simulink model "TxSteering_RxMVDR_4x4_HDL_IQ"  (R2023a)
settings: Solver=FixedStepDiscrete  StartTime=0.0  StopTime=stoptime  RelTol=1e-3
PreLoadFcn:
  | model_init
InitFcn:
  | model_init
model workspace (MAT data in the model file):
  socvcb : containers.Map (value not decoded)
values from neighbouring files (symbols this model uses):
  diagLoading = 5e-3    (= 0.005)    [model_init.m]
  dmaFIFOLength = 2^nextpow2(testSrc1.FrameLength*testSrc1.SamplesPerSymbol*2)    [model_init.m]
  fc = ConverterSampleRate*7/16    (= 860160000)    [model_init.m]
  FPGAClkRate = DataSampleRate/VectorSamplingFactor    (= 245760000)    [model_init.m]
  movavg_bitshift = nextpow2(windowSize)    [model_init.m]
  mvdrPipelineDelay = covMatDelay+movAvgDelay+matrixSolveDelay+normResponseDelay    [model_init.m]
  NCO_bits = 14    [model_init.m]
  numArrayElements = 4    [model_init.m]
  NumChan = 4    [model_init.m]
  reciprocalDelay = nextpow2(reciprocalin_dt.WordLength) + 1 + reciprocalin_dt.WordLength + 2      - strcmp(reciprocalin_dt.Signedness,'Signed') + 7    [model_init.m]
  rx_mag_delay = input_dt.WordLength + 2 + ceil(log2(NumChan)) + 1 + rx_mag_window_size    [model_init.m]
  rx_mag_inverse_delay = nextpow2(rx_mag_dt.WordLength) + 1 + rx_mag_dt.WordLength + 2 + 7    [model_init.m]
  rx_mag_sum_growth = nextpow2(rx_mag_window_size)    [model_init.m]
  rx_mag_window_size = 256    [model_init.m]
  s2mmFrameSize = testSrc1.FrameLength*testSrc1.SamplesPerSymbol*3    [model_init.m]
  testSrc1 = struct()    [model_init.m]
  testSrc2 = struct()    [model_init.m]
  windowSize = 4096    [model_init.m]
undefined symbols (not defined in the file or in its folder): Add, j, NumBits1, NumBits2, physconst, Shift
libraries: hdlsllib x29, simulink x15, embreciprocals x2, dspsrcs4 x2, dsphdlmathfun2 x1, embsystolicmatrixops x1, dsphdlsigops2 x1, commrfcorlib x1
(part 2 of 3)

== system TxSteering_RxMVDR_4x4_HDL_IQ/DUT/Rx Beamforming/MVDR HDL ==
  data_bus_in : Inport
  steering_vector : Inport  Port=2
  diag_loading : Inport  Port=3
  Compute Weight Vector : Subsystem
  Diagonal Loading : Subsystem
  Form Beam : Subsystem
  Form Covariance Matrix : Subsystem
  From Data Bus1 : Subsystem
  Moving Average : Subsystem
  Normalize Response : Subsystem
  data_bus_out : Outport
  computed_weights : Outport  Port=2
  wires:
  Normalize Response/2(wOut) -> Form Beam/3(weights), computed_weights/1
  Form Covariance Matrix/2(validOut) -> Moving Average/2(validIn)
  Compute Weight Vector/1(w) -> Normalize Response/1(wIn)
  steering_vector/1 -> Compute Weight Vector/3(steeringVector), Normalize Response/3(steeringVector)
  Form Covariance Matrix/1(dataOut) -> Moving Average/1(dataIn)
  Compute Weight Vector/2(validOut) -> Normalize Response/2(validIn)
  From Data Bus1/1(data) -> Form Covariance Matrix/1(dataIn)
  From Data Bus1/2(valid) -> Form Covariance Matrix/2(validIn)
  data_bus_in/1 -> From Data Bus1/1(bus), Form Beam/1(dataBusIn)
  Form Beam/1(dataBusOut) -> data_bus_out/1
  Normalize Response/1(wOutValid) -> Form Beam/2(weightsValid)
  Diagonal Loading/2(validOut) -> Compute Weight Vector/2(validIn)
  Moving Average/2(validOut) -> Diagonal Loading/2(validIn)
  Moving Average/1(dataOut) -> Diagonal Loading/1(dataIn)
  Diagonal Loading/1(dataOut) -> Compute Weight Vector/1(covarianceMatrix)
  diag_loading/1 -> Diagonal Loading/3(diagLoadVal)

== system TxSteering_RxMVDR_4x4_HDL_IQ/DUT/Rx Beamforming/Output Selector ==
  src_sel : Inport
  adc_data_bus : Inport  Port=2
  mvdr_in_bus : Inport  Port=3
  mvdr_out_bus : Inport  Port=4
  Delay : Delay  DelayLength=1
  Multiport Switch : MultiPortSwitch  DataPortOrder=Zero-based contiguous  zeroidx=on  SaturateOnIntegerOverflow=off  InputSameDT=off
  PackInput : Subsystem
  PackInput1 : Subsystem
  PackMVDR : Subsystem
  data_bus_out : Outport
  wires:
  Multiport Switch/1 -> Delay/1
  adc_data_bus/1 -> PackInput1/1(In1)
  mvdr_out_bus/1 -> PackMVDR/1(In1)
  mvdr_in_bus/1 -> PackInput/1(In1)
  src_sel/1 -> Multiport Switch/1
  Delay/1 -> data_bus_out/1
  PackMVDR/1(Out1) -> Multiport Switch/2
  PackInput/1(Out1) -> Multiport Switch/3
  PackInput1/1(Out1) -> Multiport Switch/4

== system TxSteering_RxMVDR_4x4_HDL_IQ/DUT/Rx Data Capture/One-Shot Capture Control ==
  validIn : Inport
  start : Inport  Port=2
  length : Inport  Port=3
  readyIn : Inport  Port=4
  AND : Logic  Inputs=3  IconShape=distinctive  AllPortsSameDT=off  OutDataTypeStr=boolean
  AND2 : Logic  IconShape=distinctive  AllPortsSameDT=off  OutDataTypeStr=boolean
  Compare To Constant : simulink/Logic and Bit Operations/Compare To Constant  relop===  const=1  OutDataTypeStr=boolean
  Compare To Zero : simulink/Logic and Bit Operations/Compare To Zero  relop=>  OutDataTypeStr=boolean
  HDL Counter : hdlsllib/Sources/HDL Counter  CountType=Free running  CountInit=0  CountStep=-1  CountMax=25  CountFromType=Initial value  CountFrom=0  CountResetPort=off  CountLoadPort=on  CountEnbPort=on  CountDirPort=off  CountHitOutputPort=off  CountDataType=Unsigned  CountWordLen=32  CountFracLen=0  CountSampTime=1
  NOT : Logic  Operator=NOT  IconShape=distinctive  AllPortsSameDT=off  OutDataTypeStr=boolean
  validOut : Outport
  lastOut : Outport  Port=2
  wires:
  HDL Counter/1 -> Compare To Constant/1, Compare To Zero/1
  Compare To Zero/1 -> NOT/1, AND/3
  AND/1 -> HDL Counter/3, validOut/1
  validIn/1 -> AND/1
  readyIn/1 -> AND/2
  length/1 -> HDL Counter/2
  AND2/1 -> HDL Counter/1
  NOT/1 -> AND2/1
  start/1 -> AND2/2
  Compare To Constant/1 -> lastOut/1

== system TxSteering_RxMVDR_4x4_HDL_IQ/DUT/Rx Data Capture/Stream FIFO ==
  dataIn : Inport
  validIn : Inport  Port=2
  lastIn : Inport  Port=3
  readyIn : Inport  Port=4
  AND : Logic  IconShape=distinctive  AllPortsSameDT=off  OutDataTypeStr=boolean
  AND1 : Logic  IconShape=distinctive  AllPortsSameDT=off  OutDataTypeStr=boolean
  Compare To Constant : simulink/Logic and Bit Operations/Compare To Constant  relop=<  const=dmaFIFOLength-1  OutDataTypeStr=boolean
  Data FIFO : hdlsllib/HDL RAMs/HDL FIFO  fifo_size=dmaFIFOLength  mode=FWFT  ratio=1  push_msg=Warning  pop_msg=Warning  show_empty=on  show_full=off  show_num=on  LabelModeActiveChoice_Mode=FWFT  rst_port=off
  Delay : Delay  DelayLength=1
  Delay1 : Delay  DelayLength=1
  Delay2 : Delay  DelayLength=1
  Last FIFO : hdlsllib/HDL RAMs/HDL FIFO  fifo_size=dmaFIFOLength  mode=FWFT  ratio=1  push_msg=Warning  pop_msg=Warning  show_empty=off  show_full=off  show_num=off  LabelModeActiveChoice_Mode=FWFT  rst_port=off
  NOT : Logic  Operator=NOT  IconShape=distinctive  AllPortsSameDT=off  OutDataTypeStr=boolean
  dataOut : Outport
  validOut : Outport  Port=2
  lastOut : Outport  Port=3
  readyOut : Outport  Port=4
  wires:
  Compare To Constant/1 -> readyOut/1
  Data FIFO/3 -> Compare To Constant/1
  [not_empty] -> AND/1
  NOT/1 -> [not_empty]
  Data FIFO/1 -> Delay/1
  Delay/1 -> dataOut/1
  readyIn/1 -> AND/2
  dataIn/1 -> Data FIFO/1
  Data FIFO/2 -> NOT/1
  validIn/1 -> Last FIFO/2, Data FIFO/2
  AND/1 -> AND1/2, Delay1/1, Data FIFO/3, Last FIFO/3
  Delay1/1 -> validOut/1
  lastIn/1 -> Last FIFO/1
  Last FIFO/1 -> AND1/1
  AND1/1 -> Delay2/1
  Delay2/1 -> lastOut/1

== system TxSteering_RxMVDR_4x4_HDL_IQ/DUT/Rx Input Preparation/Apply Calibration Coefficients ==
  Bus Element In : Inport  PortName=InBus  Element=data
  Bus Element In1 : Inport  PortName=InBus  Element=valid
  coeffIn : Inport  Port=2
  Data Type Duplicate : DataTypeDuplicate
  Data Type Conversion : DataTypeConversion  RndMeth=Convergent
  Delay : Delay  DelayLength=1
  Delay1 : Delay  DelayLength=1
  For Each Subsystem : Subsystem  TreatAsAtomicUnit=on
  Selector : Selector  InputPortWidth=4  IndexOptions=Index vector (dialog)  Indices=1  OutputSizes=1
  Bus Element Out : Outport  PortName=OutBus  Element=data
  Bus Element Out1 : Outport  PortName=OutBus  Element=valid
  wires:
  coeffIn/1 -> For Each Subsystem/3(coeffIn)
  Bus Element In/1 -> For Each Subsystem/1(dataIn), Data Type Duplicate/1
  Data Type Conversion/1 -> Delay/1, Data Type Duplicate/2
  For Each Subsystem/2(validOut) -> Selector/1
  Selector/1 -> Delay1/1
  For Each Subsystem/1(dataOut) -> Data Type Conversion/1
  Bus Element In1/1 -> For Each Subsystem/2(validIn)
  Delay/1 -> Bus Element Out/1
  Delay1/1 -> Bus Element Out1/1

== system TxSteering_RxMVDR_4x4_HDL_IQ/DUT/Rx Input Preparation/Deinterleave Complex ==
  u : Inport
  deinterleave_complex_fcn : MATLAB Function  TreatAsAtomicUnit=on
  y : Outport
  wires:
  deinterleave_complex_fcn/1(y) -> y/1
  u/1 -> deinterleave_complex_fcn/1(u)

== system TxSteering_RxMVDR_4x4_HDL_IQ/DUT/To DAC Interface/From Data Bus ==
  bus : Inport
  Bus Selector : BusSelector  OutputSignals=data,valid
  data : Outport  VectorParamsAs1DForOutWhenUnconnected=off
  valid : Outport  Port=2  VectorParamsAs1DForOutWhenUnconnected=off
  wires:
  Bus Selector/2 -> valid/1  "<valid>"
  Bus Selector/1 -> data/1  "<data>"
  bus/1 -> Bus Selector/1

== system TxSteering_RxMVDR_4x4_HDL_IQ/DUT/Tx Signal Generation/Calibration NCO ==
  note: Send the same tone to all channels
  inc : Inport
  Constant : Constant  Value=true  SampleTime=-1
  Data Type Conversion : DataTypeConversion  OutDataTypeStr=input_dt  SaturateOnIntegerOverflow=off  RndMeth=Floor
  Mux : Mux
  NCO : dsphdlsigops2/NCO  PhaseIncrementSource=Input port  PhaseIncrement=100  PhaseOffsetSource=Property  PhaseOffset=0  DitherSource=Property  NumDitherBits=4  SamplesPerFrame=1  LUTCompress=off  ResetAction=off  Waveform=Complex exponential  PhasePort=off  SimulateUsing=Code generation  AccumulatorWL=NCO_bits  PhaseQuantization=on  NumQuantizerAccumulatorBits=12  OutputDataType=Binary point scaling  OutputWL=NCO_bits  OutputFL=NCO_bits-1
  data_out : Outport
  valid_out : Outport  Port=2
  wires:
  inc/1 -> NCO/1
  NCO/2 -> valid_out/1
  Constant/1 -> NCO/2
  NCO/1 -> Data Type Conversion/1
  Data Type Conversion/1 -> Mux/1, Mux/2, Mux/3, Mux/4
  Mux/1 -> data_out/1

== system TxSteering_RxMVDR_4x4_HDL_IQ/DUT/Tx Signal Generation/Generate Steering Channels ==
  data_in : Inport  Partition=on  PartitionDimension=1  PartitionWidth=1  PartitionOffset=0
  valid_in : Inport  Port=2
  gain : Inport  Port=3  Partition=on  PartitionDimension=1  PartitionWidth=1  PartitionOffset=0
  steering_coeffs : Inport  Port=4  Partition=on  PartitionDimension=1  PartitionWidth=4  PartitionOffset=0
  Apply Gain : Subsystem
  Apply Steering Coefficients : Subsystem  TreatAsAtomicUnit=on
  Data Type Conversion : DataTypeConversion  OutDataTypeStr=fixdt(1,16,0)  SaturateOnIntegerOverflow=off  RndMeth=Floor
  For Each : ForEach  DisableCoverage=on
  Selector : Selector  InputPortWidth=4  IndexOptions=Index vector (dialog)  Indices=1  OutputSizes=1
  data_out : Outport  ConcatenationDimension=1
  valid_out : Outport  Port=2  ConcatenationDimension=1
  wires:
  Data Type Conversion/1 -> data_out/1
  Selector/1 -> valid_out/1
  steering_coeffs/1 -> Apply Steering Coefficients/3(coeff_in)
  Apply Steering Coefficients/1(data_out) -> Data Type Conversion/1
  Apply Steering Coefficients/2(valid_out) -> Selector/1
  Apply Gain/1(data_out) -> Apply Steering Coefficients/1(data_in)
  gain/1 -> Apply Gain/3(gain)
  Apply Gain/2(valid_out) -> Apply Steering Coefficients/2(valid_in)
  data_in/1 -> Apply Gain/1(data_in)
  valid_in/1 -> Apply Gain/2(valid_in)

== system TxSteering_RxMVDR_4x4_HDL_IQ/DUT/Tx Signal Generation/Sum Channels ==
  data_in : Inport
  valid_in : Inport  Port=2
  Add : Sum
  Bit Shift : hdlsllib/Logic and Bit Operations/Bit Shift  mode=Shift Right Arithmetic  N=1
  Data Type Conversion : DataTypeConversion  OutDataTypeStr=int16  SaturateOnIntegerOverflow=off  RndMeth=Floor
  Data Type Conversion1 : DataTypeConversion  OutDataTypeStr=input_dt  ConvertRealWorld=Stored Integer (SI)  SaturateOnIntegerOverflow=off  RndMeth=Floor
  Delay{,1..4} (5 alike) : Delay  DelayLength=1
  Selector : Selector  InputPortWidth=2  IndexOptions=Index vector (dialog)  Indices=1  OutputSizes=1
  Selector1 : Selector  InputPortWidth=8  IndexOptions=Index vector (dialog)  Indices=1:4  OutputSizes=1
  Selector2 : Selector  InputPortWidth=8  IndexOptions=Index vector (dialog)  Indices=5:8  OutputSizes=1
  data_out : Outport
  valid_out : Outport  Port=2
  wires:
  Bit Shift/1 -> Data Type Conversion/1
  data_in/1 -> Selector2/1, Selector1/1
  valid_in/1 -> Selector/1
  Selector/1 -> Delay3/1
  Selector2/1 -> Delay1/1
  Selector1/1 -> Delay/1
  Delay/1 -> Add/1
  Delay1/1 -> Add/2
  Delay2/1 -> Bit Shift/1
  Add/1 -> Delay2/1
  Delay3/1 -> Delay4/1
  Delay4/1 -> valid_out/1
  Data Type Conversion/1 -> Data Type Conversion1/1
  Data Type Conversion1/1 -> data_out/1

== system TxSteering_RxMVDR_4x4_HDL_IQ/DUT/Tx Signal Generation/To Data Bus ==
  data : Inport
  valid : Inport  Port=2
  Bus Creator : BusCreator  Inputs=2
  bus : Outport  VectorParamsAs1DForOutWhenUnconnected=off
  wires:
  Bus Creator/1 -> bus/1
  data/1 -> Bus Creator/1  "data"
  valid/1 -> Bus Creator/2  "valid"

== system TxSteering_RxMVDR_4x4_HDL_IQ/DUT/Tx Signal Generation/To Data Bus1 ==
  data : Inport
  valid : Inport  Port=2
  Bus Creator : BusCreator  Inputs=2
  bus : Outport  VectorParamsAs1DForOutWhenUnconnected=off
  wires:
  valid/1 -> Bus Creator/2  "valid"
  data/1 -> Bus Creator/1  "data"
  Bus Creator/1 -> bus/1

== system TxSteering_RxMVDR_4x4_HDL_IQ/DUT/Tx Signal Generation/Tx Source LUT ==
  Constant : Constant  Value=true  SampleTime=-1
  Delay : Delay  DelayLength=1
  HDL Counter : hdlsllib/Sources/HDL Counter  CountType=Count limited  CountInit=0  CountStep=1  CountMax=length(testSrc1.Data)-1  CountFromType=Initial value  CountFrom=0  CountResetPort=off  CountLoadPort=off  CountEnbPort=off  CountDirPort=off  CountHitOutputPort=off  CountDataType=Unsigned  CountWordLen=nextpow2(length(testSrc1.Data))  CountFracLen=0  CountSampTime=1/FPGAClkRate
  HDL Counter1 : hdlsllib/Sources/HDL Counter  CountType=Count limited  CountInit=0  CountStep=1  CountMax=length(testSrc2.Data)-1  CountFromType=Initial value  CountFrom=0  CountResetPort=off  CountLoadPort=off  CountEnbPort=off  CountDirPort=off  CountHitOutputPort=off  CountDataType=Unsigned  CountWordLen=nextpow2(length(testSrc2.Data))  CountFracLen=0  CountSampTime=1/FPGAClkRate
  HW Delay : UnitDelay  SampleTime=-1  HasFrameUpgradeWarning=on
  HW Delay1 : UnitDelay  SampleTime=-1  HasFrameUpgradeWarning=on
  Mux : Mux  Inputs=2
  Source 1 LUT : LookupNDDirect  NumberOfTableDimensions=1  Table=testSrc1.Data  DiagnosticForOutOfRangeInput=Error  TableDataTypeStr=fixdt(1,16,15)
  Source 2 LUT : LookupNDDirect  NumberOfTableDimensions=1  Table=testSrc2.Data  DiagnosticForOutOfRangeInput=Error  TableDataTypeStr=fixdt(1,16,15)
  data_out : Outport
  valid_out : Outport  Port=2
  wires:
  Source 1 LUT/1 -> HW Delay/1
  HDL Counter/1 -> Source 1 LUT/1
  Source 2 LUT/1 -> HW Delay1/1
  HW Delay/1 -> Mux/1
  HW Delay1/1 -> Mux/2
  Mux/1 -> data_out/1
  Constant/1 -> Delay/1
  Delay/1 -> valid_out/1
  HDL Counter1/1 -> Source 2 LUT/1

== system TxSteering_RxMVDR_4x4_HDL_IQ/S2MM DMA Behavioral/Unpack to uint32/Enabled Subsystem ==
  dataIn : Inport
  Enable : EnablePort
  Extract Bits : simulink/Logic and Bit Operations/Extract Bits  bitsToExtract=Range of bits  numBits=8  bitIdxRange=[0 31]  outScalingMode=Treat bit field as an integer
  Extract Bits1 : simulink/Logic and Bit Operations/Extract Bits  bitsToExtract=Range of bits  numBits=8  bitIdxRange=[32 63]  outScalingMode=Treat bit field as an integer
  Extract Bits2 : simulink/Logic and Bit Operations/Extract Bits  bitsToExtract=Range of bits  numBits=8  bitIdxRange=[64 95]  outScalingMode=Treat bit field as an integer
  Extract Bits3 : simulink/Logic and Bit Operations/Extract Bits  bitsToExtract=Range of bits  numBits=8  bitIdxRange=[96 127]  outScalingMode=Treat bit field as an integer
  Matrix Concatenate : Concatenate  NumInputs=4  Mode=Multidimensional array
  Reshape : Reshape  OutputDimensionality=Row vector (2-D)
  Reshape1 : Reshape
  dataOut : Outport
  wires:
  dataIn/1 -> Reshape/1
  Extract Bits/1 -> Matrix Concatenate/1
  Extract Bits3/1 -> Matrix Concatenate/4
  Extract Bits2/1 -> Matrix Concatenate/3
  Extract Bits1/1 -> Matrix Concatenate/2
  Reshape/1 -> Extract Bits/1, Extract Bits1/1, Extract Bits2/1, Extract Bits3/1
  Matrix Concatenate/1 -> Reshape1/1
  Reshape1/1 -> dataOut/1

== system TxSteering_RxMVDR_4x4_HDL_IQ/Software Interface Behavioral/GenSteeringCoeffs Rx/Interleave Complex 3 ==
  u : Inport
  interleave_complex_fcn : MATLAB Function  TreatAsAtomicUnit=on
  y : Outport
  wires:
  interleave_complex_fcn/1(y) -> y/1
  u/1 -> interleave_complex_fcn/1(u)

== system TxSteering_RxMVDR_4x4_HDL_IQ/Software Interface Behavioral/GenSteeringCoeffs Tx Source 1/Interleave Complex 3 ==
  u : Inport
  interleave_complex_fcn : MATLAB Function  TreatAsAtomicUnit=on
  y : Outport
  wires:
  interleave_complex_fcn/1(y) -> y/1
  u/1 -> interleave_complex_fcn/1(u)

== system TxSteering_RxMVDR_4x4_HDL_IQ/Software Interface Behavioral/GenSteeringCoeffs Tx Source 2/Interleave Complex 3 ==
  u : Inport
  interleave_complex_fcn : MATLAB Function  TreatAsAtomicUnit=on
  y : Outport
  wires:
  interleave_complex_fcn/1(y) -> y/1
  u/1 -> interleave_complex_fcn/1(u)

== system TxSteering_RxMVDR_4x4_HDL_IQ/DUT/Rx Beamforming/Input Gate/From Data Bus ==
  bus : Inport
  Bus Selector : BusSelector  OutputSignals=data,valid
  data : Outport  VectorParamsAs1DForOutWhenUnconnected=off
  valid : Outport  Port=2  VectorParamsAs1DForOutWhenUnconnected=off
  wires:
  Bus Selector/2 -> valid/1  "<valid>"
  Bus Selector/1 -> data/1  "<data>"
  bus/1 -> Bus Selector/1

== system TxSteering_RxMVDR_4x4_HDL_IQ/DUT/Rx Beamforming/Input Gate/To Data Bus1 ==
  data : Inport
  valid : Inport  Port=2
  Bus Creator : BusCreator  Inputs=2
  bus : Outport  VectorParamsAs1DForOutWhenUnconnected=off
  wires:
  Bus Creator/1 -> bus/1
  data/1 -> Bus Creator/1  "data"
  valid/1 -> Bus Creator/2  "valid"

== system TxSteering_RxMVDR_4x4_HDL_IQ/DUT/Rx Beamforming/Input Scaling/Compute Input Magnitude ==
  data_in : Inport
  valid_in : Inport  Port=2
  Add1 : Sum  Inputs=++-  AccumDataTypeStr=fixdt(1,17+rx_mag_sum_growth,15)  OutDataTypeStr=Inherit: Same as accumulator
  Bit Shift : hdlsllib/Logic and Bit Operations/Bit Shift  mode=Shift Right Arithmetic  N=nextpow2(NumChan)
  Bit Shift1 : hdlsllib/Logic and Bit Operations/Bit Shift  mode=Shift Right Arithmetic  N=rx_mag_sum_growth
  Complex to Magnitude-Angle : dsphdlmathfun2/Complex to Magnitude-Angle  NumIterationsSource=Auto  NumIterations=10  OutputFormat=Magnitude  AngleFormat=Normalized  ScaleOutput=on  ScalingMethod=Shift-Add  SimulateUsing=Code generation
  Data Type Conversion : DataTypeConversion  OutDataTypeStr=rx_mag_dt  RndMeth=Convergent  SaturateOnIntegerOverflow=off
  Data Type Conversion1 : DataTypeConversion  OutDataTypeStr=rx_mag_dt  SaturateOnIntegerOverflow=off  RndMeth=Floor
  Data Type Conversion2 : DataTypeConversion  OutDataTypeStr=rx_mag_dt  SaturateOnIntegerOverflow=off  RndMeth=Floor
  Delay Enabled Synchronous : Subsystem  mask(Delay Enabled){DelayLength=rx_mag_window_size, InitialCondition=0.0}
      mask prompts: DelayLength "Simulink:blkprm_prompts:DelayBlkDelayLength"; InitialCondition "Simulink:blkprm_prompts:DelayBlkInitCond"
      mask help: Implements a delay with synchronous enable.
      mask TypeOptions DelayLength: Synchronous Delay/Delay/DelayLength
      mask TypeOptions InitialCondition: Synchronous Delay/Delay/InitialCondition
      mask DialogControl DelayLength Prompt: Delay length:
      mask DialogControl InitialCondition Prompt: Initial condition:
      mask Display:
      | port_label('input', 1, 'u');
      | port_label('input', 2, 'E');
      | text(0.45,0.45, 'Z');
      | DelayLengthStr = get_param(gcbh,'DelayLength');
      | try
      |     DelayLength = evalin('base',DelayLengthStr);
      |     text(0.55,0.55, sprintf('-%d',DelayLength));
      | catch ME
      |     text(0.55,0.55, '-N');
      | end
  Delay1 : Delay  DelayLength=1
  Delay2 : Delay  DelayLength=1
  Delay3 : Delay  DelayLength=ceil(log2(NumChan))
  Tree Sum : Subsystem
  Unit Delay Enabled Synchronous : hdlsllib/Discrete/Unit Delay Enabled Synchronous  InitialCondition=0.0  SampleTime=-1
  Wait for Running Sum Init : Subsystem
  mag : Outport
  mag_valid : Outport  Port=2
  wires:
  Delay1/1 -> Add1/2, Delay Enabled Synchronous/1(u)
  Unit Delay Enabled Synchronous/1 -> Add1/1, Bit Shift1/1
  Tree Sum/1(Out1) -> Bit Shift/1
  Bit Shift/1 -> Data Type Conversion/1
  Data Type Conversion/1 -> Delay1/1
  Delay2/1 -> Delay Enabled Synchronous/2(E), Unit Delay Enabled Synchronous/2, Wait for Running Sum Init/1(In1)
  Complex to Magnitude-Angle/1 -> Data Type Conversion2/1
  Bit Shift1/1 -> Data Type Conversion1/1
  valid_in/1 -> Complex to Magnitude-Angle/2
  Delay3/1 -> Delay2/1
  Add1/1 -> Unit Delay Enabled Synchronous/1
  Delay Enabled Synchronous/1(y) -> Add1/3
  data_in/1 -> Complex to Magnitude-Angle/1
  Complex to Magnitude-Angle/2 -> Delay3/1
  Data Type Conversion2/1 -> Tree Sum/1(In1)
  Data Type Conversion1/1 -> mag/1  "RxMag"
  Wait for Running Sum Init/1(mag1) -> mag_valid/1  "RxMagValid"

== system TxSteering_RxMVDR_4x4_HDL_IQ/DUT/Rx Beamforming/Input Scaling/Compute Magnitude Inverse Scale ==
  mag_in : Inport
  mag_valid : Inport  Port=2
  Bit Shift1 : hdlsllib/Logic and Bit Operations/Bit Shift  mode=Shift Right Arithmetic  N=1
  Data Type Conversion : DataTypeConversion  OutDataTypeStr=rx_gain_dt  SaturateOnIntegerOverflow=off  RndMeth=Floor
  Real Reciprocal HDL Optimized : embreciprocals/Real Reciprocal HDL Optimized  OutputType=rx_mag_inv_dt
      settings: LibrarySourceBlock=embeddedMatrixLib/Math Operations/Real Reciprocal HDL Optimized
  Unit Delay Enabled Synchronous : hdlsllib/Discrete/Unit Delay Enabled Synchronous  InitialCondition=0.0  SampleTime=-1
  scale_out : Outport
  wires:
  mag_in/1 -> Real Reciprocal HDL Optimized/1
  mag_valid/1 -> Real Reciprocal HDL Optimized/2
  Real Reciprocal HDL Optimized/1 -> Bit Shift1/1
  Real Reciprocal HDL Optimized/2 -> Unit Delay Enabled Synchronous/2
  Unit Delay Enabled Synchronous/1 -> scale_out/1
  Bit Shift1/1 -> Data Type Conversion/1
  Data Type Conversion/1 -> Unit Delay Enabled Synchronous/1

== system TxSteering_RxMVDR_4x4_HDL_IQ/DUT/Rx Beamforming/MVDR HDL/Compute Weight Vector ==
  covarianceMatrix : Inport
  validIn : Inport  Port=2
  steeringVector : Inport  Port=3
  Complex Partial-Systolic Matrix Solve Using QR Decomposition : embsystolicmatrixops/Complex Partial-Systolic Matrix Solve Using QR Decomposition  m=4  n=4  p=1  regularizationParameter=0  OutputType=matrixdivbacksub_dt
  Constant : Constant  Value=false  SampleTime=-1
  Data Type Conversion2 : DataTypeConversion  OutDataTypeStr=matrixdivin_dt  SaturateOnIntegerOverflow=off  RndMeth=Floor
  Deserialize Output Data : Subsystem
  Reshape1 : Reshape  OutputDimensionality=Column vector (2-D)  OutputDimensions=[4,4]
  Serialize Input Data : Subsystem
  w : Outport
  validOut : Outport  Port=2
  wires:
  steeringVector/1 -> Data Type Conversion2/1
  Data Type Conversion2/1 -> Reshape1/1
  validIn/1 -> Serialize Input Data/3(validIn)
  Constant/1 -> Complex Partial-Systolic Matrix Solve Using QR Decomposition/4
  Serialize Input Data/3(validOut) -> Complex Partial-Systolic Matrix Solve Using QR Decomposition/3  "matrixSolveValidIn"
  Complex Partial-Systolic Matrix Solve Using QR Decomposition/3 -> Serialize Input Data/4(readyIn)  "matrixSolveReady"
  Serialize Input Data/1(AOut) -> Complex Partial-Systolic Matrix Solve Using QR Decomposition/1
  Reshape1/1 -> Serialize Input Data/2(BIn)
  Complex Partial-Systolic Matrix Solve Using QR Decomposition/1 -> Deserialize Output Data/1(dataIn)
  Complex Partial-Systolic Matrix Solve Using QR Decomposition/2 -> Deserialize Output Data/2(validIn)  "matrixSolveValidOut"
  Deserialize Output Data/1(dataOut) -> w/1
  Deserialize Output Data/2(validOut) -> validOut/1
  Serialize Input Data/2(BOut) -> Complex Partial-Systolic Matrix Solve Using QR Decomposition/2
  covarianceMatrix/1 -> Serialize Input Data/1(AIn)

== system TxSteering_RxMVDR_4x4_HDL_IQ/DUT/Rx Beamforming/MVDR HDL/Diagonal Loading ==
  dataIn : Inport
  validIn : Inport  Port=2
  diagLoadVal : Inport  Port=3
  Add : Sum
  Data Type Conversion1 : DataTypeConversion  OutDataTypeStr=matrixdivin_dt  SaturateOnIntegerOverflow=off  RndMeth=Floor
  Delay3 : Delay  DelayLength=1
  Delay6 : Delay  DelayLength=1
  Generate Loading Eye Matrix : MATLAB Function  TreatAsAtomicUnit=on
  Reshape1 : Reshape  OutputDimensions=[4,4]
  To Workspace2 : ToWorkspace  VariableName=Ecx_loaded  SampleTime=-1
      settings: Save2DSignal=2-D array (concatenate along first dimension)
  dataOut : Outport
  validOut : Outport  Port=2
  wires:
  Reshape1/1 -> To Workspace2/1
  Data Type Conversion1/1 -> dataOut/1, Reshape1/1
  Delay3/1 -> Data Type Conversion1/1
  dataIn/1 -> Add/2
  Generate Loading Eye Matrix/1(out) -> Add/1
  Add/1 -> Delay3/1
  Delay6/1 -> validOut/1
  diagLoadVal/1 -> Generate Loading Eye Matrix/1(in)
  validIn/1 -> Delay6/1

== system TxSteering_RxMVDR_4x4_HDL_IQ/DUT/Rx Beamforming/MVDR HDL/Form Beam ==
  Bus Element In : Inport  PortName=dataBusIn  Element=data
  Bus Element In1 : Inport  PortName=dataBusIn  Element=valid
  weightsValid : Inport  Port=2
  weights : Inport  Port=3
  AND : Logic  IconShape=distinctive  AllPortsSameDT=off  OutDataTypeStr=boolean
  Data Type Conversion : DataTypeConversion  OutDataTypeStr=output_dt  SaturateOnIntegerOverflow=off  RndMeth=Floor
  Delay1 : Delay  DelayLength=6
  Delay2 : Delay
  Delay3 : Delay  DelayLength=mvdrPipelineDelay
  Delay7 : Delay  DelayLength=mvdrPipelineDelay
  Math Function2 : Math  Operator=conj
  Parallel Complex Multiply : Subsystem  TreatAsAtomicUnit=on
  Reshape : Reshape
  Reshape1 : Reshape
  Rx Beam - Spectrum : SpectrumAnalyzer  WindowPosition=[145.000000,315.000000,771.000000,515.000000,]  ScopeFrameLocation=window  Method=Welch  SampleRateSource=Property  SampleRate=DataSampleRate  AxesScaling=Manual  Span=245760000  StartFrequency=-122880000  StopFrequency=122880000  WindowLength=32  AveragingMethod=Exponential  YLimits=[-29.86220698,5.27402686]
      settings: OpenAtSimulationStart=off
  Tree Sum : Subsystem
  Bus Element Out : Outport  PortName=dataBusOut  Element=data
  Out Bus Element : Outport  PortName=dataBusOut  Element=valid
  wires:
  Parallel Complex Multiply/1(z) -> Tree Sum/1(In1)
  Tree Sum/1(Out1) -> Data Type Conversion/1
  Math Function2/1 -> Reshape/1
  weights/1 -> Math Function2/1
  Reshape/1 -> Parallel Complex Multiply/2(z2)
  Reshape1/1 -> Parallel Complex Multiply/1(z1)
  Data Type Conversion/1 -> Rx Beam - Spectrum/1, Bus Element Out/1
  Delay2/1 -> Out Bus Element/1
  Delay1/1 -> Delay2/1
  Bus Element In1/1 -> Delay3/1
  Bus Element In/1 -> Delay7/1
  Delay7/1 -> Reshape1/1
  Delay3/1 -> AND/1
  weightsValid/1 -> AND/2
  AND/1 -> Delay1/1

== system TxSteering_RxMVDR_4x4_HDL_IQ/DUT/Rx Beamforming/MVDR HDL/Form Covariance Matrix ==
  dataIn : Inport
  validIn : Inport  Port=2
  Conj : Math  Operator=conj  SaturateOnIntegerOverflow=off
  Data Type Conversion : DataTypeConversion  OutDataTypeStr=covmat_dt  SaturateOnIntegerOverflow=off  RndMeth=Floor
  Data Type Conversion1 : DataTypeConversion  OutDataTypeStr=adc_dt  SaturateOnIntegerOverflow=off  RndMeth=Floor
  Delay : Delay  DelayLength=6
  Matrix Multiply Partitioned : Subsystem  TreatAsAtomicUnit=on
  Reshape : Reshape
  dataOut : Outport
  validOut : Outport  Port=2
  wires:
  validIn/1 -> Delay/1
  dataIn/1 -> Data Type Conversion1/1
  Reshape/1 -> Conj/1, Matrix Multiply Partitioned/1(x)  "x"
  Matrix Multiply Partitioned/1(C) -> Data Type Conversion/1  "x * x'"
  Delay/1 -> validOut/1
  Conj/1 -> Matrix Multiply Partitioned/2(x_conj)
  Data Type Conversion1/1 -> Reshape/1
  Data Type Conversion/1 -> dataOut/1

== system TxSteering_RxMVDR_4x4_HDL_IQ/DUT/Rx Beamforming/MVDR HDL/From Data Bus1 ==
  bus : Inport
  Bus Selector : BusSelector  OutputSignals=data,valid
  data : Outport
  valid : Outport  Port=2
  wires:
  bus/1 -> Bus Selector/1
  Bus Selector/1 -> data/1  "<data>"
  Bus Selector/2 -> valid/1  "<valid>"

== system TxSteering_RxMVDR_4x4_HDL_IQ/DUT/Rx Beamforming/MVDR HDL/Moving Average ==
  note: Shift replaces gain by 1/sqrt(windowSize)
  dataIn : Inport
  validIn : Inport  Port=2
  Add1 : Sum  Inputs=++-  AccumDataTypeStr=movavg_accum_dt  OutDataTypeStr=Inherit: Same as accumulator
  Bit Shift : hdlsllib/Logic and Bit Operations/Bit Shift  mode=Shift Right Arithmetic  N=movavg_bitshift
  Data Type Conversion : DataTypeConversion  OutDataTypeStr=movavg_out_dt  SaturateOnIntegerOverflow=off  RndMeth=Floor
  Delay{2..5} (4 alike) : Delay  DelayLength=1
  Reshape : Reshape  OutputDimensionality=Customize  OutputDimensions=[4,4]
  Reshape1 : Reshape  OutputDimensions=[4,4]
  Reshape2 : Reshape  OutputDimensions=[4,4]
  To Workspace : ToWorkspace  VariableName=Ecx  SampleTime=-1
      settings: Save2DSignal=2-D array (concatenate along first dimension)
  To Workspace1 : ToWorkspace  VariableName=Ecx_valid  SampleTime=-1
      settings: Save2DSignal=2-D array (concatenate along first dimension)
  To Workspace2 : ToWorkspace  VariableName=Ecx_scaled  SampleTime=-1
      settings: Save2DSignal=2-D array (concatenate along first dimension)
  To Workspace3 : ToWorkspace  VariableName=Ecx_scaled_valid  SampleTime=-1
      settings: Save2DSignal=2-D array (concatenate along first dimension)
  Unit Delay Enabled Synchronous : hdlsllib/Discrete/Unit Delay Enabled Synchronous  InitialCondition=0.0  SampleTime=-1
  Wait for Running Sum Init : Subsystem
  Window Delay : Subsystem
  dataOut : Outport
  validOut : Outport  Port=2
  wires:
  Bit Shift/1 -> Data Type Conversion/1
  Unit Delay Enabled Synchronous/1 -> Bit Shift/1, Add1/1, Reshape2/1  "Ecx"
  Add1/1 -> Unit Delay Enabled Synchronous/1
  dataIn/1 -> Delay2/1
  validIn/1 -> Delay3/1
  Delay2/1 -> Reshape1/1
  Delay4/1 -> dataOut/1
  Delay5/1 -> validOut/1
  Delay3/1 -> Window Delay/2(E), Unit Delay Enabled Synchronous/2, Wait for Running Sum Init/1(In1)
  Wait for Running Sum Init/1(Out1) -> To Workspace1/1, To Workspace3/1, Delay5/1  "Ecx_valid"
  Data Type Conversion/1 -> To Workspace2/1, Reshape/1
  Reshape/1 -> Delay4/1
  Reshape1/1 -> Window Delay/1(u), Add1/2
  Window Delay/1(y) -> Add1/3
  Reshape2/1 -> To Workspace/1

== system TxSteering_RxMVDR_4x4_HDL_IQ/DUT/Rx Beamforming/MVDR HDL/Normalize Response ==
  note: This subsystem scales the weight vector to ensure unit gain in the target direction.
  wIn : Inport
  validIn : Inport  Port=2
  steeringVector : Inport  Port=3
  MVDR Weight Update : Subsystem
  Set Latch : Subsystem
  Unit Delay Enabled Synchronous : hdlsllib/Discrete/Unit Delay Enabled Synchronous  InitialCondition=0.0  SampleTime=-1
  wOutValid : Outport
  wOut : Outport  Port=2
  wires:
  steeringVector/1 -> MVDR Weight Update/1(sv)
  wIn/1 -> MVDR Weight Update/2(wp)
  MVDR Weight Update/1(w) -> Unit Delay Enabled Synchronous/1
  MVDR Weight Update/2(validOut) -> Set Latch/1(S), Unit Delay Enabled Synchronous/2
  Unit Delay Enabled Synchronous/1 -> wOut/1
  validIn/1 -> MVDR Weight Update/3(validIn)
  Set Latch/1(Q) -> wOutValid/1

== system TxSteering_RxMVDR_4x4_HDL_IQ/DUT/Rx Beamforming/Output Selector/PackInput ==
  In1 : Inport
  Bus Creator : BusCreator  Inputs=2
  Bus Selector : BusSelector  OutputSignals=data,valid
  Pack Samples : Subsystem  mask(Pack Samples){is_complex=on}
      mask prompts: is_complex "Input is complex"
      mask help:
      | Pack data samples to unsigned word.
      |
      | The first vector element is placed in the LSB, and the last vector element is placed in the MSB.
      |
      | For complex inputs, real and imaginary components are interleaved, with real component starting in LSB position.
      mask Display: fprintf('Pack\nSamples');
  Out1 : Outport
  wires:
  Pack Samples/1(y) -> Bus Creator/1  "data"
  Bus Selector/1 -> Pack Samples/1(u)  "<data>"
  Bus Selector/2 -> Bus Creator/2  "<valid>"
  Bus Creator/1 -> Out1/1
  In1/1 -> Bus Selector/1

== system TxSteering_RxMVDR_4x4_HDL_IQ/DUT/Rx Beamforming/Output Selector/PackInput1 ==
  In1 : Inport
  Bus Creator : BusCreator  Inputs=2
  Bus Selector : BusSelector  OutputSignals=data,valid
  Pack Samples : Subsystem  mask(Pack Samples){is_complex=on}
      mask prompts: is_complex "Input is complex"
      mask help:
      | Pack data samples to unsigned word.
      |
      | The first vector element is placed in the LSB, and the last vector element is placed in the MSB.
      |
      | For complex inputs, real and imaginary components are interleaved, with real component starting in LSB position.
      mask Display: fprintf('Pack\nSamples');
  Out1 : Outport
  wires:
  In1/1 -> Bus Selector/1
  Bus Creator/1 -> Out1/1
  Bus Selector/2 -> Bus Creator/2  "<valid>"
  Bus Selector/1 -> Pack Samples/1(u)  "<data>"
  Pack Samples/1(y) -> Bus Creator/1  "data"

== system TxSteering_RxMVDR_4x4_HDL_IQ/DUT/Rx Beamforming/Output Selector/PackMVDR ==
  In1 : Inport
  Bus Creator : BusCreator  Inputs=2
  Bus Selector : BusSelector  OutputSignals=data,valid
  Data Type Conversion1 : DataTypeConversion  OutDataTypeStr=fixdt(0,128,0)  SaturateOnIntegerOverflow=off  RndMeth=Floor
  Pack Samples : Subsystem  mask(Pack Samples){is_complex=on}
      mask prompts: is_complex "Input is complex"
      mask help:
      | Pack data samples to unsigned word.
      |
      | The first vector element is placed in the LSB, and the last vector element is placed in the MSB.
      |
      | For complex inputs, real and imaginary components are interleaved, with real component starting in LSB position.
      mask Display: fprintf('Pack\nSamples');
  Out1 : Outport
  wires:
  Pack Samples/1(y) -> Data Type Conversion1/1
  Data Type Conversion1/1 -> Bus Creator/1  "data"
  Bus Selector/2 -> Bus Creator/2  "<valid>"
  In1/1 -> Bus Selector/1
  Bus Creator/1 -> Out1/1
  Bus Selector/1 -> Pack Samples/1(u)  "<data>"

== system TxSteering_RxMVDR_4x4_HDL_IQ/DUT/Rx Input Preparation/Apply Calibration Coefficients/For Each Subsystem ==
  dataIn : Inport  Partition=on  PartitionDimension=2  PartitionWidth=1  PartitionOffset=0
  validIn : Inport  Port=2
  coeffIn : Inport  Port=3  Partition=on  PartitionDimension=1  PartitionWidth=1  PartitionOffset=0
  Delay : Delay  DelayLength=6
  For Each : ForEach  DisableCoverage=on
  HDL Complex Multiply : Subsystem  mask(HDL Complex Multiplier (3 Multiply, 5 Add)){D1=2, D2=1, D3=1, D4=1, D5=1}
      mask help:
      | Xilinx devices:
      | - Set D1 = 1 or 2 to trade off speed & FF resources
      | - Set D2-D5 = 1 to fully leverage DSP48 pipelines
      | - Use sync reset
      |
      | Intel FPGAs:
      | - Set D1 = 1 or 2 depending on device family
      | - Set D5 = 1; D2, D3, D4 = 0
      | - Use async reset
      mask init:
      | delay = D1+D2+D3+D4+D5;
      mask Display:
      | fprintf('Pipelined\nComplex Multiply\nLatency=%d',delay);
      | port_label('input',1,'z1');
      | port_label('input',2,'z2');
  dataOut : Outport  ConcatenationDimension=2
  validOut : Outport  Port=2  ConcatenationDimension=1
  wires:
  Delay/1 -> validOut/1
  HDL Complex Multiply/1(Out1) -> dataOut/1
  validIn/1 -> Delay/1
  coeffIn/1 -> HDL Complex Multiply/2(In2)
  dataIn/1 -> HDL Complex Multiply/1(In1)

== system TxSteering_RxMVDR_4x4_HDL_IQ/DUT/Tx Signal Generation/Generate Steering Channels/Apply Gain ==
  data_in : Inport
  valid_in : Inport  Port=2
  gain : Inport  Port=3
  Data Type Duplicate : DataTypeDuplicate
  Data Type Conversion1 : DataTypeConversion  SaturateOnIntegerOverflow=off  RndMeth=Floor
  Data Type Conversion2 : DataTypeConversion  OutDataTypeStr=int16  ConvertRealWorld=Stored Integer (SI)  SaturateOnIntegerOverflow=off  RndMeth=Floor  LockScale=on
  PipelineDelay : Delay  DelayLength=1
  PipelineDelay1 : Delay  DelayLength=1
  PipelineDelay2 : Delay
  PipelineDelay3 : Delay  DelayLength=1
  PipelineDelay4 : Delay
  Product : Product
  data_out : Outport
  valid_out : Outport  Port=2  VectorParamsAs1DForOutWhenUnconnected=off
  wires:
  data_in/1 -> Data Type Conversion2/1
  gain/1 -> PipelineDelay/1
  PipelineDelay/1 -> Product/1
  PipelineDelay1/1 -> Product/2
  Product/1 -> PipelineDelay2/1
  PipelineDelay2/1 -> Data Type Conversion1/1
  Data Type Conversion1/1 -> data_out/1, Data Type Duplicate/2
  Data Type Conversion2/1 -> Data Type Duplicate/1, PipelineDelay1/1
  valid_in/1 -> PipelineDelay3/1
  PipelineDelay3/1 -> PipelineDelay4/1
  PipelineDelay4/1 -> valid_out/1

== system TxSteering_RxMVDR_4x4_HDL_IQ/DUT/Tx Signal Generation/Generate Steering Channels/Apply Steering Coefficients ==
  data_in : Inport
  valid_in : Inport  Port=2
  coeff_in : Inport  Port=3  Partition=on  PartitionDimension=1  PartitionWidth=1  PartitionOffset=0
  For Each : ForEach  DisableCoverage=on
  HDL Complex Multiplier : Subsystem
  data_out : Outport  ConcatenationDimension=1
  valid_out : Outport  Port=2  ConcatenationDimension=1
  wires:
  data_in/1 -> HDL Complex Multiplier/1(z1)
  coeff_in/1 -> HDL Complex Multiplier/2(z2)
  valid_in/1 -> HDL Complex Multiplier/3(validIn)
  HDL Complex Multiplier/1(z) -> data_out/1
  HDL Complex Multiplier/2(validOut) -> valid_out/1

== system TxSteering_RxMVDR_4x4_HDL_IQ/DUT/Rx Beamforming/Input Scaling/Compute Input Magnitude/Delay Enabled Synchronous ==
  u : Inport
  E : Inport  Port=2
  Synchronous Delay : Subsystem
  y : Outport
  wires:
  u/1 -> Synchronous Delay/1(u)
  E/1 -> Synchronous Delay/2(E)
  Synchronous Delay/1(y) -> y/1

== system TxSteering_RxMVDR_4x4_HDL_IQ/DUT/Rx Beamforming/Input Scaling/Compute Input Magnitude/Tree Sum ==
  In1 : Inport
  Add : Sum
  Add1 : Sum
  Add2 : Sum
  Delay1 : Delay  DelayLength=1
  Delay2 : Delay  DelayLength=1
  Delay3 : Delay  DelayLength=1
  Demux : Demux
  Out1 : Outport
  wires:
  In1/1 -> Demux/1
  Demux/1 -> Add/1
  Demux/2 -> Add/2
  Add/1 -> Delay3/1
  Add1/1 -> Delay1/1
  Demux/3 -> Add1/1
  Demux/4 -> Add1/2
  Delay3/1 -> Add2/1
  Delay1/1 -> Add2/2
  Add2/1 -> Delay2/1
  Delay2/1 -> Out1/1

== system TxSteering_RxMVDR_4x4_HDL_IQ/DUT/Rx Beamforming/Input Scaling/Compute Input Magnitude/Wait for Running Sum Init ==
  In1 : Inport
  Compare To Constant : simulink/Logic and Bit Operations/Compare To Constant  relop=<  const=rx_mag_window_size  OutDataTypeStr=boolean
  HDL Counter : hdlsllib/Sources/HDL Counter  CountType=Free running  CountInit=0  CountStep=1  CountMax=25  CountFromType=Initial value  CountFrom=0  CountResetPort=off  CountLoadPort=off  CountEnbPort=on  CountDirPort=off  CountHitOutputPort=off  CountDataType=Unsigned  CountWordLen=nextpow2(rx_mag_window_size)+1  CountFracLen=0  CountSampTime=1
  Logical Operator : Logic  IconShape=distinctive  AllPortsSameDT=off  OutDataTypeStr=boolean
  Logical Operator1 : Logic  IconShape=distinctive  AllPortsSameDT=off  OutDataTypeStr=boolean
  Logical Operator2 : Logic  Operator=NOT  IconShape=distinctive  AllPortsSameDT=off  OutDataTypeStr=boolean
  mag1 : Outport
  wires:
  Logical Operator2/1 -> Logical Operator/2
  Logical Operator1/1 -> HDL Counter/1
  Compare To Constant/1 -> Logical Operator1/2, Logical Operator2/1
  Logical Operator/1 -> mag1/1
  HDL Counter/1 -> Compare To Constant/1
  In1/1 -> Logical Operator1/1, Logical Operator/1

== system TxSteering_RxMVDR_4x4_HDL_IQ/DUT/Rx Beamforming/MVDR HDL/Compute Weight Vector/Deserialize Output Data ==
  dataIn : Inport
  validIn : Inport  Port=2
  AND : Logic  IconShape=distinctive  AllPortsSameDT=off  OutDataTypeStr=boolean
  Assignment : Assignment  IndexMode=Zero-based  DiagnosticForDimensions=Warning  IndexOptions=Index vector (port)  Indices=1  OutputSizes=4
  Compare To Constant : simulink/Logic and Bit Operations/Compare To Constant  relop===  const=3.0  OutDataTypeStr=boolean
  Data Type Duplicate : DataTypeDuplicate
  Data Type Conversion : DataTypeConversion  OutDataTypeStr=uint8  SaturateOnIntegerOverflow=off  RndMeth=Floor
  Data Type Conversion4 : DataTypeConversion  OutDataTypeStr=matrixdivout_dt  RndMeth=Convergent  SaturateOnIntegerOverflow=off
  Delay{,1..3} (4 alike) : Delay  DelayLength=1
  HDL Counter : hdlsllib/Sources/HDL Counter  CountType=Free running  CountInit=0  CountStep=1  CountMax=25  CountFromType=Initial value  CountFrom=0  CountResetPort=off  CountLoadPort=off  CountEnbPort=on  CountDirPort=off  CountHitOutputPort=off  CountDataType=Unsigned  CountWordLen=2  CountFracLen=0  CountSampTime=1
  To Workspace : ToWorkspace  VariableName=wp  SampleTime=-1
      settings: Save2DSignal=2-D array (concatenate along first dimension)
  To Workspace1 : ToWorkspace  VariableName=wp_valid  SampleTime=-1
      settings: Save2DSignal=2-D array (concatenate along first dimension)
  To Workspace3 : ToWorkspace  VariableName=matrix_solve_X_out  SampleTime=-1
      settings: Save2DSignal=2-D array (concatenate along first dimension)
  To Workspace4 : ToWorkspace  VariableName=matrix_solve_valid_out  SampleTime=-1
      settings: Save2DSignal=2-D array (concatenate along first dimension)
  Unit Delay Enabled Synchronous : hdlsllib/Discrete/Unit Delay Enabled Synchronous  InitialCondition=complex(zeros(4,1))  SampleTime=-1
  Unit Delay Enabled Synchronous1 : hdlsllib/Discrete/Unit Delay Enabled Synchronous  InitialCondition=0  SampleTime=-1
  dataOut : Outport
  validOut : Outport  Port=2
  wires:
  AND/1 -> Delay/1
  HDL Counter/1 -> Compare To Constant/1, Data Type Conversion/1
  dataIn/1 -> Data Type Conversion4/1, To Workspace3/1
  Compare To Constant/1 -> AND/1
  Delay/1 -> Delay1/1, Unit Delay Enabled Synchronous1/2
  Data Type Conversion/1 -> Assignment/3
  validIn/1 -> To Workspace4/1, Delay3/1
  Assignment/1 -> Unit Delay Enabled Synchronous/1
  Unit Delay Enabled Synchronous/1 -> Assignment/1, Data Type Duplicate/2, Unit Delay Enabled Synchronous1/1
  Delay1/1 -> To Workspace1/1, validOut/1
  Unit Delay Enabled Synchronous1/1 -> dataOut/1, To Workspace/1
  Data Type Conversion4/1 -> Delay2/1
  Delay2/1 -> Data Type Duplicate/1, Assignment/2
  Delay3/1 -> HDL Counter/1, Unit Delay Enabled Synchronous/2, AND/2

== system TxSteering_RxMVDR_4x4_HDL_IQ/DUT/Rx Beamforming/MVDR HDL/Compute Weight Vector/Serialize Input Data ==
  AIn : Inport
  BIn : Inport  Port=2
  validIn : Inport  Port=3
  readyIn : Inport  Port=4
  AND : Logic  IconShape=distinctive  AllPortsSameDT=off  OutDataTypeStr=boolean
  Compare To Constant : simulink/Logic and Bit Operations/Compare To Constant  relop===  const=0  OutDataTypeStr=boolean
  Detect Rise Positive : simulink/Logic and Bit Operations/Detect Rise Positive  vinit=0  OutDataTypeStr=boolean
  HDL Counter : hdlsllib/Sources/HDL Counter  CountType=Free running  CountInit=0  CountStep=1  CountMax=25  CountFromType=Initial value  CountFrom=0  CountResetPort=off  CountLoadPort=off  CountEnbPort=on  CountDirPort=off  CountHitOutputPort=off  CountDataType=Unsigned  CountWordLen=2  CountFracLen=0  CountSampTime=1
  Output Selector : Subsystem
  Output Selector1 : Subsystem
  To Workspace : ToWorkspace  VariableName=matrix_in_latch  SampleTime=-1
      settings: Save2DSignal=2-D array (concatenate along first dimension)
  To Workspace1 : ToWorkspace  VariableName=matrix_solve_valid_in  SampleTime=-1
      settings: Save2DSignal=2-D array (concatenate along first dimension)
  To Workspace2 : ToWorkspace  VariableName=matrix_solve_A_in  SampleTime=-1
      settings: Save2DSignal=2-D array (concatenate along first dimension)
  To Workspace3 : ToWorkspace  VariableName=matrix_solve_B_in  SampleTime=-1
      settings: Save2DSignal=2-D array (concatenate along first dimension)
  Unit Delay : UnitDelay  SampleTime=-1  HasFrameUpgradeWarning=on
  Unit Delay Enabled Synchronous1 : hdlsllib/Discrete/Unit Delay Enabled Synchronous  InitialCondition=0.0  SampleTime=-1
  Unit Delay Enabled Synchronous2 : hdlsllib/Discrete/Unit Delay Enabled Synchronous  InitialCondition=0.0  SampleTime=-1
  readyQueue : MATLAB Function  TreatAsAtomicUnit=on
  AOut : Outport
  BOut : Outport  Port=2
  validOut : Outport  Port=3
  wires:
  readyIn/1 -> Detect Rise Positive/1
  HDL Counter/1 -> Compare To Constant/1, Output Selector1/1(idx), Output Selector/1(idx)
  Compare To Constant/1 -> AND/1
  readyQueue/1(validOut) -> HDL Counter/1, AND/2, To Workspace1/1, validOut/1
  Detect Rise Positive/1 -> readyQueue/1(readyEdge)
  AIn/1 -> Unit Delay Enabled Synchronous1/1
  validIn/1 -> Unit Delay Enabled Synchronous2/2, Unit Delay Enabled Synchronous1/2, Unit Delay/1
  Unit Delay/1 -> readyQueue/2(validIn)
  BIn/1 -> Unit Delay Enabled Synchronous2/1
  AND/1 -> To Workspace/1, Output Selector1/2(first), Output Selector/2(first)  "matrix_in_latch"
  Unit Delay Enabled Synchronous1/1 -> Output Selector/3(dataIn)
  Output Selector/1(dataOut) -> To Workspace2/1, AOut/1
  Unit Delay Enabled Synchronous2/1 -> Output Selector1/3(dataIn)
  Output Selector1/1(dataOut) -> To Workspace3/1, BOut/1

== system TxSteering_RxMVDR_4x4_HDL_IQ/DUT/Rx Beamforming/MVDR HDL/Form Beam/Parallel Complex Multiply ==
  z1 : Inport  Partition=on  PartitionDimension=1  PartitionWidth=1  PartitionOffset=0
  z2 : Inport  Port=2  Partition=on  PartitionDimension=1  PartitionWidth=1  PartitionOffset=0
  For Each : ForEach  DisableCoverage=on
  HDL Complex Multiply : Subsystem  mask(HDL Complex Multiplier (3 Multiply, 5 Add)){D1=2, D2=1, D3=1, D4=1, D5=1}
      mask help:
      | Xilinx devices:
      | - Set D1 = 1 or 2 to trade off speed & FF resources
      | - Set D2-D5 = 1 to fully leverage DSP48 pipelines
      | - Use sync reset
      |
      | Intel FPGAs:
      | - Set D1 = 1 or 2 depending on device family
      | - Set D5 = 1; D2, D3, D4 = 0
      | - Use async reset
      mask init:
      | delay = D1+D2+D3+D4+D5;
      mask Display:
      | fprintf('Delay=%d',delay);
      | port_label('input',1,'z1');
      | port_label('input',2,'z2');
  z : Outport  ConcatenationDimension=1
  wires:
  z1/1 -> HDL Complex Multiply/1(In1)
  z2/1 -> HDL Complex Multiply/2(In2)
  HDL Complex Multiply/1(Out1) -> z/1

== system TxSteering_RxMVDR_4x4_HDL_IQ/DUT/Rx Beamforming/MVDR HDL/Form Beam/Tree Sum ==
  In1 : Inport
  Delay3 : Delay  DelayLength=ceil(log2(numArrayElements))
  Tree Sum of Elements : Sum  Inputs=+  OutDataTypeStr=Inherit: Same as first input  LockScale=on
  Out1 : Outport
  wires:
  Delay3/1 -> Out1/1
  In1/1 -> Tree Sum of Elements/1
  Tree Sum of Elements/1 -> Delay3/1

== system TxSteering_RxMVDR_4x4_HDL_IQ/DUT/Rx Beamforming/MVDR HDL/Form Covariance Matrix/Matrix Multiply Partitioned ==
  x : Inport
  x_conj : Inport  Port=2
  Partition x_conj : Subsystem
  Reshape : Reshape  OutputDimensionality=Customize  OutputDimensions=[4,4]
  C : Outport
  wires:
  x/1 -> Partition x_conj/1(x)
  x_conj/1 -> Partition x_conj/2(x_conj)
  Partition x_conj/1(C) -> Reshape/1
  Reshape/1 -> C/1

== system TxSteering_RxMVDR_4x4_HDL_IQ/DUT/Rx Beamforming/MVDR HDL/Moving Average/Wait for Running Sum Init ==
  In1 : Inport
  Compare To Constant : simulink/Logic and Bit Operations/Compare To Constant  relop=<  const=windowSize  OutDataTypeStr=boolean
  HDL Counter : hdlsllib/Sources/HDL Counter  CountType=Free running  CountInit=0  CountStep=1  CountMax=25  CountFromType=Initial value  CountFrom=0  CountResetPort=off  CountLoadPort=off  CountEnbPort=on  CountDirPort=off  CountHitOutputPort=off  CountDataType=Unsigned  CountWordLen=nextpow2(windowSize)+1  CountFracLen=0  CountSampTime=1
  Logical Operator : Logic  IconShape=distinctive  AllPortsSameDT=off  OutDataTypeStr=boolean
  Logical Operator1 : Logic  IconShape=distinctive  AllPortsSameDT=off  OutDataTypeStr=boolean
  Logical Operator2 : Logic  Operator=NOT  IconShape=distinctive  AllPortsSameDT=off  OutDataTypeStr=boolean
  Out1 : Outport
  wires:
  Logical Operator2/1 -> Logical Operator/2
  Logical Operator1/1 -> HDL Counter/1
  Compare To Constant/1 -> Logical Operator1/2, Logical Operator2/1
  Logical Operator/1 -> Out1/1
  HDL Counter/1 -> Compare To Constant/1
  In1/1 -> Logical Operator1/1, Logical Operator/1

== system TxSteering_RxMVDR_4x4_HDL_IQ/DUT/Rx Beamforming/MVDR HDL/Moving Average/Window Delay ==
  u : Inport
  E : Inport  Port=2
  Delay Enabled Synchronous RAM Based : Subsystem  mask{delay=windowSize-1}
      mask prompts: delay "Delay length:"
      mask init:
      | addrWidth = max(nextpow2(delay),4);
      | 
      | blk=gcb;
      | add_blk = [blk '/Add'];
      | Simulink.suppressDiagnostic(add_blk,'SimulinkFixedPoint:util:Overflowoccurred');
      mask Display:
      | blkh=gcbh;
      | delay_val = get_param(gcb,'delay');
      | try
      |     val = num2str(evalin('base',delay_val));
      | catch ME
      |     val = 'd';
      | end
      | 
      | text(0.5,0.5,['z^{-' val '}'],'texmode','on');
      | 
      | port_label('input',1,'u');
      | port_label('input',2,'E');
      | 
      | color('blue');
      | text(0.65,0.9,'RAM')
  Unit Delay Enabled Synchronous : hdlsllib/Discrete/Unit Delay Enabled Synchronous  InitialCondition=0.0  SampleTime=-1
  y : Outport
  wires:
  E/1 -> Unit Delay Enabled Synchronous/2, Delay Enabled Synchronous RAM Based/2(E)
  u/1 -> Delay Enabled Synchronous RAM Based/1(u)
  Delay Enabled Synchronous RAM Based/1(y) -> Unit Delay Enabled Synchronous/1
  Unit Delay Enabled Synchronous/1 -> y/1

== system TxSteering_RxMVDR_4x4_HDL_IQ/DUT/Rx Beamforming/MVDR HDL/Normalize Response/MVDR Weight Update ==
  sv : Inport
  wp : Inport  Port=2
  validIn : Inport  Port=3
  Delay{,1,3..6} (6 alike) : Delay  DelayLength=1
  Delay2 : Delay  DelayLength=9
  Inner Product : Subsystem
  Vector / Scalar Divide : Subsystem
  w : Outport
  validOut : Outport  Port=2
  wires:
  wp/1 -> Delay3/1
  Vector / Scalar Divide/1(w) -> w/1
  Delay4/1 -> Inner Product/1(sv)
  Inner Product/1(y) -> Delay5/1
  Delay6/1 -> Vector / Scalar Divide/1(x)
  Delay/1 -> Vector / Scalar Divide/3(validIn)
  sv/1 -> Delay4/1
  Delay3/1 -> Delay2/1, Inner Product/2(wp)
  Delay5/1 -> Vector / Scalar Divide/2(y)
  Inner Product/2(validOut) -> Delay/1
  validIn/1 -> Delay1/1
  Vector / Scalar Divide/2(validOut) -> validOut/1
  Delay1/1 -> Inner Product/3(validIn)
  Delay2/1 -> Delay6/1
